simulink model "total_senario"  (R2019a)
settings: Solver=ode4  StartTime=0.0  StopTime=40  FixedStep=0.001  RelTol=1e-3
libraries: nesl_utility x16, sm_lib x13, simulink x1
(part 2 of 3)

== matlab function total_senario/SMC/MATLAB Function ==
  data: q input; u output; qd input; Dqd input; D2qd input
function u = fcn(q, qd, Dqd, D2qd)

c = 10;
k = 100;

L1 = 0.3; L2 = 0.4; L3 = 0.08;
c1 =  c; c2 = c; c3 = c; c4 = c;
k1 = k; k2 = k; k3 = k; k4 = k;
m1 = 4; m2 = 3; m3 = 1;

% s1 = 0;
% s2 = 0;
% s3 = 0;
% s4 = 0;

% SMC
e1 = qd(1) - q(1);
e2 = Dqd(1) - q(2);

e3 = qd(2) - q(3);
e4 = Dqd(2) - q(4);

e5 = qd(3) - q(5);
e6 = Dqd(3) - q(6);

e7 = qd(4) - q(7);
e8 = Dqd(4) - q(8);



s1 = c1*e1 + e2 ;
s2 = c2*e3 + e4 ;
s3 = c3*e5 + e6 ;
s4 = c4*e7 + e8 ;

%sgn
% if s1 > 0
%     sgn1 = 1;
% elseif s1 == 0
%     sgn1 = 0;
% elseif s1 < 0  
%     sgn1 = -1;
% end

% if s2 > 0
%     sgn2 = 1;
% elseif s2 == 0
%     sgn2 = 0;
% elseif s2 < 0  
%     sgn2 = -1;
% end

% if s3 > 0
%     sgn3 = 1;
% elseif s3 == 0
%     sgn3 = 0;
% elseif s3 < 0  
%     sgn3 = -1;
% end

% if s4 > 0
%     sgn4 = 1;
% elseif s4 == 0
%     sgn4 = 0;
% elseif s4 < 0  
%     sgn4 = -1;
% end

%sat
if abs(s1) <= 1
    sgn1 = s1;
elseif s1 > 1
    sgn1 = 1;
else
    sgn1 = -1;
end

if abs(s2) <= 1
    sgn2 = s2;
elseif s2 > 1
    sgn2 = 1;
else
    sgn2 = -1;
end

if abs(s3) <= 1
    sgn3 = s3;
elseif s3 > 1
    sgn3 = 1;
else
    sgn3 = -1;
end

if abs(s4) <= 1
    sgn4 = s4;
elseif s4 > 1
    sgn4 = 1;
else
    sgn4 = -1;
end

npsii = q(1);
ndpsii = q(2);
nth1 = q(3);
ndth1 = q(4);
nth2 = q(5);
ndth2 = q(6);
nth3 = q(7);
ndth3 = q(8);

%dynamcis
V = [- L3^2*m3*ndpsii*ndth1*sin(2*nth1 + 2*nth2 + 2*nth3) - L3^2*m3*ndpsii*ndth2*sin(2*nth1 + 2*nth2 + 2*nth3) - L3^2*m3*ndpsii*ndth3*sin(2*nth1 + 2*nth2 + 2*nth3) - L1^2*m1*ndpsii*ndth1*sin(2*nth1) - L1^2*m2*ndpsii*ndth1*sin(2*nth1) - L1^2*m3*ndpsii*ndth1*sin(2*nth1) - L2^2*m2*ndpsii*ndth1*sin(2*nth1 + 2*nth2) - L2^2*m2*ndpsii*ndth2*sin(2*nth1 + 2*nth2) - L2^2*m3*ndpsii*ndth1*sin(2*nth1 + 2*nth2) - L2^2*m3*ndpsii*ndth2*sin(2*nth1 + 2*nth2) - 2*L2*L3*m3*ndpsii*ndth1*sin(2*nth1 + 2*nth2 + nth3) - 2*L2*L3*m3*ndpsii*ndth2*sin(2*nth1 + 2*nth2 + nth3) - L2*L3*m3*ndpsii*ndth3*sin(2*nth1 + 2*nth2 + nth3) - L1*L2*m2*ndpsii*ndth2*sin(nth2) - L1*L2*m3*ndpsii*ndth2*sin(nth2) - L2*L3*m3*ndpsii*ndth3*sin(nth3) - 2*L1*L2*m2*ndpsii*ndth1*sin(2*nth1 + nth2) - L1*L2*m2*ndpsii*ndth2*sin(2*nth1 + nth2) - 2*L1*L2*m3*ndpsii*ndth1*sin(2*nth1 + nth2) - L1*L2*m3*ndpsii*ndth2*sin(2*nth1 + nth2) - 2*L1*L3*m3*ndpsii*ndth1*sin(2*nth1 + nth2 + nth3) - L1*L3*m3*ndpsii*ndth2*sin(2*nth1 + nth2 + nth3) - L1*L3*m3*ndpsii*ndth3*sin(2*nth1 + nth2 + nth3) - L1*L3*m3*ndpsii*ndth2*sin(nth2 + nth3) - L1*L3*m3*ndpsii*ndth3*sin(nth2 + nth3);
                                                                                                                                                                                                                                                                               (L3^2*m3*ndpsii^2*sin(2*nth1 + 2*nth2 + 2*nth3))/2 + (L1^2*m1*ndpsii^2*sin(2*nth1))/2 + (L1^2*m2*ndpsii^2*sin(2*nth1))/2 + (L1^2*m3*ndpsii^2*sin(2*nth1))/2 + (L2^2*m2*ndpsii^2*sin(2*nth1 + 2*nth2))/2 + (L2^2*m3*ndpsii^2*sin(2*nth1 + 2*nth2))/2 + L2*L3*m3*ndpsii^2*sin(2*nth1 + 2*nth2 + nth3) - L1*L2*m2*ndth2^2*sin(nth2) - L1*L2*m3*ndth2^2*sin(nth2) - L2*L3*m3*ndth3^2*sin(nth3) + L1*L2*m2*ndpsii^2*sin(2*nth1 + nth2) + L1*L2*m3*ndpsii^2*sin(2*nth1 + nth2) + L1*L3*m3*ndpsii^2*sin(2*nth1 + nth2 + nth3) - L1*L3*m3*ndth2^2*sin(nth2 + nth3) - L1*L3*m3*ndth3^2*sin(nth2 + nth3) - 2*L1*L2*m2*ndth1*ndth2*sin(nth2) - 2*L1*L2*m3*ndth1*ndth2*sin(nth2) - 2*L2*L3*m3*ndth1*ndth3*sin(nth3) - 2*L2*L3*m3*ndth2*ndth3*sin(nth3) - 2*L1*L3*m3*ndth1*ndth2*sin(nth2 + nth3) - 2*L1*L3*m3*ndth1*ndth3*sin(nth2 + nth3) - 2*L1*L3*m3*ndth2*ndth3*sin(nth2 + nth3);
                                                                                                                                                                                                                                                                                                                                                                                                                                                                                                       (L3^2*m3*ndpsii^2*sin(2*nth1 + 2*nth2 + 2*nth3))/2 + (L2^2*m2*ndpsii^2*sin(2*nth1 + 2*nth2))/2 + (L2^2*m3*ndpsii^2*sin(2*nth1 + 2*nth2))/2 + L2*L3*m3*ndpsii^2*sin(2*nth1 + 2*nth2 + nth3) + (L1*L2*m2*ndpsii^2*sin(nth2))/2 + (L1*L2*m3*ndpsii^2*sin(nth2))/2 + L1*L2*m2*ndth1^2*sin(nth2) + L1*L2*m3*ndth1^2*sin(nth2) - L2*L3*m3*ndth3^2*sin(nth3) + (L1*L2*m2*ndpsii^2*sin(2*nth1 + nth2))/2 + (L1*L2*m3*ndpsii^2*sin(2*nth1 + nth2))/2 + (L1*L3*m3*ndpsii^2*sin(2*nth1 + nth2 + nth3))/2 + (L1*L3*m3*ndpsii^2*sin(nth2 + nth3))/2 + L1*L3*m3*ndth1^2*sin(nth2 + nth3) - 2*L2*L3*m3*ndth1*ndth3*sin(nth3) - 2*L2*L3*m3*ndth2*ndth3*sin(nth3);
                                                                                                                                                                                                                                                                                                                                                                                                                                                                                                                                                                      (L3*m3*(L1*ndpsii^2*sin(nth2 + nth3) + 2*L1*ndth1^2*sin(nth2 + nth3) + L2*ndpsii^2*sin(2*nth1 + 2*nth2 + nth3) + L2*ndpsii^2*sin(nth3) + 2*L2*ndth1^2*sin(nth3) + 2*L2*ndth2^2*sin(nth3) + L3*ndpsii^2*sin(2*nth1 + 2*nth2 + 2*nth3) + L1*ndpsii^2*sin(2*nth1 + nth2 + nth3) + 2*L1*ndth1*ndth2*sin(nth2 + nth3) + 2*L1*ndth1*ndth3*sin(nth2 + nth3) + 4*L2*ndth1*ndth2*sin(nth3) + 2*L2*ndth1*ndth3*sin(nth3) + 2*L2*ndth2*ndth3*sin(nth3)))/2 - L3*m3*(L1*ndth1*ndth2*sin(nth2 + nth3) + L1*ndth1*ndth3*sin(nth2 + nth3) + L2*ndth1*ndth3*sin(nth3) + L2*ndth2*ndth3*sin(nth3))];
%
G = 9.81*[                                                                                                                                    0;
L3*m3*cos(nth1 + nth2 + nth3) + L2*m2*cos(nth1 + nth2) + L2*m3*cos(nth1 + nth2) + L1*m1*cos(nth1) + L1*m2*cos(nth1) + L1*m3*cos(nth1);
                                                      L3*m3*cos(nth1 + nth2 + nth3) + L2*m2*cos(nth1 + nth2) + L2*m3*cos(nth1 + nth2);
                                                                                                        L3*m3*cos(nth1 + nth2 + nth3)];
%
M = [[(L1^2*m1)/2 + (L1^2*m2)/2 + (L1^2*m3)/2 + (L2^2*m2)/2 + (L2^2*m3)/2 + (L3^2*m3)/2 + (L3^2*m3*cos(2*nth1 + 2*nth2 + 2*nth3))/2 + (L1^2*m1*cos(2*nth1))/2 + (L1^2*m2*cos(2*nth1))/2 + (L1^2*m3*cos(2*nth1))/2 + (L2^2*m2*cos(2*nth1 + 2*nth2))/2 + (L2^2*m3*cos(2*nth1 + 2*nth2))/2 + L1*L3*m3*cos(nth2 + nth3) + L2*L3*m3*cos(2*nth1 + 2*nth2 + nth3) + L1*L2*m2*cos(nth2) + L1*L2*m3*cos(nth2) + L2*L3*m3*cos(nth3) + L1*L2*m2*cos(2*nth1 + nth2) + L1*L2*m3*cos(2*nth1 + nth2) + L1*L3*m3*cos(2*nth1 + nth2 + nth3),                                                                                                                                                            0,                                                                                                                        0,                                                        0];
[                                                                                                                                                                                                                                                                                                                                                                                                                                                                                                                   0, L1^2*m1 + L1^2*m2 + L1^2*m3 + L2^2*m2 + L2^2*m3 + L3^2*m3 + 2*L1*L3*m3*cos(nth2 + nth3) + 2*L1*L2*m2*cos(nth2) + 2*L1*L2*m3*cos(nth2) + 2*L2*L3*m3*cos(nth3), L2^2*m2 + L2^2*m3 + L3^2*m3 + L1*L3*m3*cos(nth2 + nth3) + L1*L2*m2*cos(nth2) + L1*L2*m3*cos(nth2) + 2*L2*L3*m3*cos(nth3), L3^2*m3 + L1*L3*m3*cos(nth2 + nth3) + L2*L3*m3*cos(nth3)];
[                                                                                                                                                                                                                                                                                                                                                                                                                                                                                                                   0,                                     L2^2*m2 + L2^2*m3 + L3^2*m3 + L1*L3*m3*cos(nth2 + nth3) + L1*L2*m2*cos(nth2) + L1*L2*m3*cos(nth2) + 2*L2*L3*m3*cos(nth3),                                                                       L2^2*m2 + L2^2*m3 + L3^2*m3 + 2*L2*L3*m3*cos(nth3),                             m3*L3^2 + L2*m3*cos(nth3)*L3];
[                                                                                                                                                                                                                                                                                                                                                                                                                                                                                                                   0,                                                                                                              L3*m3*(L3 + L1*cos(nth2 + nth3) + L2*cos(nth3)),                                                                                                L3*m3*(L3 + L2*cos(nth3)),                                                  L3^2*m3]];
%

N = V + G;

F = -pinv(M)*N ;

% X(1) = psi, X(3) = th1, X(5) = th2, X(7) = th3
tau1_hat = c1*e2 + D2qd(1) - F(1) + k1*sgn1 ;
tau2_hat = c2*e4 + D2qd(2) - F(2) + k2*sgn2 ;
tau3_hat = c3*e6 + D2qd(3) - F(3) + k3*sgn3 ;
tau4_hat = c4*e8 + D2qd(4) - F(4) + k4*sgn4 ;

Tau_hat = [tau1_hat;tau2_hat;tau3_hat;tau4_hat];

u = M*[tau1_hat;tau2_hat;tau3_hat;tau4_hat] ;
% tau1 = u(1) ;
% tau2 = u(2) ;
% tau3 = u(3) ;
% tau4 = u(4) ;

% x_ddt = pinv(M)*(Tau_hat - N) ;
% x_ddt = pinv(M)*(Tau - N) ;


% if abs(e1*e2) < 0.05
%     t_reg1 = t;
% else
%     t_reg1 = 0;
% end
% 
% if abs(e3*e4) < 0.05
%     t_reg2 = t;
% else
%     t_reg2 = 0;
% end
% 
% if abs(e5*e6) < 0.05
%     t_reg3 = t;
% else
%     t_reg3 = 0;
% end
% 
% if abs(e7*e8) < 0.05
%     t_reg4 = t;
% else
%     t_reg4 = 0;
% end

% dXdt = [X(2); x_ddt(1) ; X(4); x_ddt(2); X(6); x_ddt(3); X(8); x_ddt(4) ] ;
end


%%%%%%%%%%%%%%%%%%%%%%%%%%%%%%%%%%%%%%%%%%%%%%%%%%%%%%%%%%%%%%%%%%%%%%%%%%%%%%%%%%%%%%%%%%%%%%%%
% function u = fcn(q, qd, Dqd, D2qd)
% u = zeros(4, 1);
% 
% % parameter
% g = 9.81;
% m1 = 4;
% m2 = 3;
% m3 = 1;
% L1 = 0.4;
% L2 = 0.3;
% L3 = 0.08;
% 
% npsii = q(1);
% nth1 = q(2);
% nth2 = q(3);
% nth3 = q(4);
% ndpsii = q(5);
% ndth1 = q(6);
% ndth2 = q(7);
% ndth3 = q(8);
% 
% 
% M11 = (L1^2*m1)/2 + (L1^2*m2)/2 + (L1^2*m3)/2 + (L2^2*m2)/2 + (L2^2*m3)/2 + (L3^2*m3)/2 + (L3^2*m3*cos(2*nth1 + 2*nth2 + 2*nth3))/2 + (L1^2*m1*cos(2*nth1))/2 + (L1^2*m2*cos(2*nth1))/2 + (L1^2*m3*cos(2*nth1))/2 + (L2^2*m2*cos(2*nth1 + 2*nth2))/2 + (L2^2*m3*cos(2*nth1 + 2*nth2))/2 + L1*L3*m3*cos(nth2 + nth3) + L2*L3*m3*cos(2*nth1 + 2*nth2 + nth3) + L1*L2*m2*cos(nth2) + L1*L2*m3*cos(nth2) + L2*L3*m3*cos(nth3) + L1*L2*m2*cos(2*nth1 + nth2) + L1*L2*m3*cos(2*nth1 + nth2) + L1*L3*m3*cos(2*nth1 + nth2 + nth3);
% M12 = 0;
% M13 = 0;
% M14 = 0;
% 
% M21 = 0;
% M22 = L1^2*m1 + L1^2*m2 + L1^2*m3 + L2^2*m2 + L2^2*m3 + L3^2*m3 + 2*L1*L3*m3*cos(nth2 + nth3) + 2*L1*L2*m2*cos(nth2) + 2*L1*L2*m3*cos(nth2) + 2*L2*L3*m3*cos(nth3);
% M23 = L2^2*m2 + L2^2*m3 + L3^2*m3 + L1*L3*m3*cos(nth2 + nth3) + L1*L2*m2*cos(nth2) + L1*L2*m3*cos(nth2) + 2*L2*L3*m3*cos(nth3);
% M24 = L3^2*m3 + L1*L3*m3*cos(nth2 + nth3) + L2*L3*m3*cos(nth3);
% 
% M31 = 0;
% M32 = L2^2*m2 + L2^2*m3 + L3^2*m3 + L1*L3*m3*cos(nth2 + nth3) + L1*L2*m2*cos(nth2) + L1*L2*m3*cos(nth2) + 2*L2*L3*m3*cos(nth3);
% M33 = L2^2*m2 + L2^2*m3 + L3^2*m3 + 2*L2*L3*m3*cos(nth3);
% M34 = m3*L3^2 + L2*m3*cos(nth3)*L3;
% 
% M41 = 0;
% M42 = L3*m3*(L3 + L1*cos(nth2 + nth3) + L2*cos(nth3));
% M43 = L3*m3*(L3 + L2*cos(nth3));
% M44 = L3^2*m3;
% 
% M = [M11 M12 M13 M14; M21 M22 M23 M24 ;M31 M32 M33 M34 ;M41 M42 M43 M44];
% 
% % coriolis vector, [V]
% V1 = -L3^2*m3*ndpsii*ndth1*sin(2*nth1 + 2*nth2 + 2*nth3) - L3^2*m3*ndpsii*ndth2*sin(2*nth1 + 2*nth2 + 2*nth3) - L3^2*m3*ndpsii*ndth3*sin(2*nth1 + 2*nth2 + 2*nth3) - L1^2*m1*ndpsii*ndth1*sin(2*nth1) - L1^2*m2*ndpsii*ndth1*sin(2*nth1) - L1^2*m3*ndpsii*ndth1*sin(2*nth1) - L2^2*m2*ndpsii*ndth1*sin(2*nth1 + 2*nth2) - L2^2*m2*ndpsii*ndth2*sin(2*nth1 + 2*nth2) - L2^2*m3*ndpsii*ndth1*sin(2*nth1 + 2*nth2) - L2^2*m3*ndpsii*ndth2*sin(2*nth1 + 2*nth2) - 2*L2*L3*m3*ndpsii*ndth1*sin(2*nth1 + 2*nth2 + nth3) - 2*L2*L3*m3*ndpsii*ndth2*sin(2*nth1 + 2*nth2 + nth3) - L2*L3*m3*ndpsii*ndth3*sin(2*nth1 + 2*nth2 + nth3) - L1*L2*m2*ndpsii*ndth2*sin(nth2) - L1*L2*m3*ndpsii*ndth2*sin(nth2) - L2*L3*m3*ndpsii*ndth3*sin(nth3) - 2*L1*L2*m2*ndpsii*ndth1*sin(2*nth1 + nth2) - L1*L2*m2*ndpsii*ndth2*sin(2*nth1 + nth2) - 2*L1*L2*m3*ndpsii*ndth1*sin(2*nth1 + nth2) - L1*L2*m3*ndpsii*ndth2*sin(2*nth1 + nth2) - 2*L1*L3*m3*ndpsii*ndth1*sin(2*nth1 + nth2 + nth3) - L1*L3*m3*ndpsii*ndth2*sin(2*nth1 + nth2 + nth3) - L1*L3*m3*ndpsii*ndth3*sin(2*nth1 + nth2 + nth3) - L1*L3*m3*ndpsii*ndth2*sin(nth2 + nth3) - L1*L3*m3*ndpsii*ndth3*sin(nth2 + nth3);
% V2 = (L3^2*m3*ndpsii^2*sin(2*nth1 + 2*nth2 + 2*nth3))/2 + (L1^2*m1*ndpsii^2*sin(2*nth1))/2 + (L1^2*m2*ndpsii^2*sin(2*nth1))/2 + (L1^2*m3*ndpsii^2*sin(2*nth1))/2 + (L2^2*m2*ndpsii^2*sin(2*nth1 + 2*nth2))/2 + (L2^2*m3*ndpsii^2*sin(2*nth1 + 2*nth2))/2 + L2*L3*m3*ndpsii^2*sin(2*nth1 + 2*nth2 + nth3) - L1*L2*m2*ndth2^2*sin(nth2) - L1*L2*m3*ndth2^2*sin(nth2) - L2*L3*m3*ndth3^2*sin(nth3) + L1*L2*m2*ndpsii^2*sin(2*nth1 + nth2) + L1*L2*m3*ndpsii^2*sin(2*nth1 + nth2) + L1*L3*m3*ndpsii^2*sin(2*nth1 + nth2 + nth3) - L1*L3*m3*ndth2^2*sin(nth2 + nth3) - L1*L3*m3*ndth3^2*sin(nth2 + nth3) - 2*L1*L2*m2*ndth1*ndth2*sin(nth2) - 2*L1*L2*m3*ndth1*ndth2*sin(nth2) - 2*L2*L3*m3*ndth1*ndth3*sin(nth3) - 2*L2*L3*m3*ndth2*ndth3*sin(nth3) - 2*L1*L3*m3*ndth1*ndth2*sin(nth2 + nth3) - 2*L1*L3*m3*ndth1*ndth3*sin(nth2 + nth3) - 2*L1*L3*m3*ndth2*ndth3*sin(nth2 + nth3);
% V3 = (L3^2*m3*ndpsii^2*sin(2*nth1 + 2*nth2 + 2*nth3))/2 + (L2^2*m2*ndpsii^2*sin(2*nth1 + 2*nth2))/2 + (L2^2*m3*ndpsii^2*sin(2*nth1 + 2*nth2))/2 + L2*L3*m3*ndpsii^2*sin(2*nth1 + 2*nth2 + nth3) + (L1*L2*m2*ndpsii^2*sin(nth2))/2 + (L1*L2*m3*ndpsii^2*sin(nth2))/2 + L1*L2*m2*ndth1^2*sin(nth2) + L1*L2*m3*ndth1^2*sin(nth2) - L2*L3*m3*ndth3^2*sin(nth3) + (L1*L2*m2*ndpsii^2*sin(2*nth1 + nth2))/2 + (L1*L2*m3*ndpsii^2*sin(2*nth1 + nth2))/2 + (L1*L3*m3*ndpsii^2*sin(2*nth1 + nth2 + nth3))/2 + (L1*L3*m3*ndpsii^2*sin(nth2 + nth3))/2 + L1*L3*m3*ndth1^2*sin(nth2 + nth3) - 2*L2*L3*m3*ndth1*ndth3*sin(nth3) - 2*L2*L3*m3*ndth2*ndth3*sin(nth3);
% V4 = (L3*m3*(L1*ndpsii^2*sin(nth2 + nth3) + 2*L1*ndth1^2*sin(nth2 + nth3) + L2*ndpsii^2*sin(2*nth1 + 2*nth2 + nth3) + L2*ndpsii^2*sin(nth3) + 2*L2*ndth1^2*sin(nth3) + 2*L2*ndth2^2*sin(nth3) + L3*ndpsii^2*sin(2*nth1 + 2*nth2 + 2*nth3) + L1*ndpsii^2*sin(2*nth1 + nth2 + nth3) + 2*L1*ndth1*ndth2*sin(nth2 + nth3) + 2*L1*ndth1*ndth3*sin(nth2 + nth3) + 4*L2*ndth1*ndth2*sin(nth3) + 2*L2*ndth1*ndth3*sin(nth3) + 2*L2*ndth2*ndth3*sin(nth3)))/2 - L3*m3*(L1*ndth1*ndth2*sin(nth2 + nth3) + L1*ndth1*ndth3*sin(nth2 + nth3) + L2*ndth1*ndth3*sin(nth3) + L2*ndth2*ndth3*sin(nth3));
% 
% V = [V1; V2; V3; V4];
% 
% % gravity vector, [G]
% G1 = 0;
% G2 = g*(L3*m3*cos(nth1 + nth2 + nth3) + L2*m2*cos(nth1 + nth2) + L2*m3*cos(nth1 + nth2) + L1*m1*cos(nth1) + L1*m2*cos(nth1) + L1*m3*cos(nth1));
% G3 = g*(L3*m3*cos(nth1 + nth2 + nth3) + L2*m2*cos(nth1 + nth2) + L2*m3*cos(nth1 + nth2));
% G4 = L3*g*m3*cos(nth1 + nth2 + nth3);
% 
% G = [G1; G2; G3; G4];
% 
% % SMC
% e1 = qd(1) - q(1);
% e2 = qd(2) - q(2);
% e3 = qd(3) - q(3);
% e4 = qd(4) - q(4);
% 
% e5 = Dqd(1) - q(5);
% e6 = Dqd(2) - q(6);
% e7 = Dqd(3) - q(7);
% e8 = Dqd(4) - q(8);
% 
% % [C] matrix
% c1 = 5;
% c2 = 5;
% c3 = 5;
% c4 = 5;
% C = diag([c1, c2, c3, c4]);
% 
% % sliding line
% s = [e5; e6; e7; e8] + C*[e1; e2; e3; e4];
% 
% % design [Q], [K]
% del1 = 0.005*10^4;
% del2 = 0.005*10^4;
% del3 = 0.005*10^4;
% del4 = 0.005*10^4;
% 
% A = M\eye(size(M));
% w1max = abs(A(1, 1))*del1 + abs(A(1, 2))*del2 + abs(A(1, 3))*del3 + abs(A(1,4))*del4;
% w2max = abs(A(2, 1))*del1 + abs(A(2, 2))*del2 + abs(A(2, 3))*del3 + abs(A(2,4))*del4;
% w3max = abs(A(3, 1))*del1 + abs(A(3, 2))*del2 + abs(A(3, 3))*del3 + abs(A(3,4))*del4;
% w4max = abs(A(4, 1))*del1 + abs(A(4, 2))*del2 + abs(A(4, 3))*del3 + abs(A(4,4))*del4;
% 
% k1 = 5;
% k2 = 5;
% k3 = 5;
% k4 = 5;
% 
% Q1 = -k1 - w1max;
% Q2 = -k2 - w2max;
% Q3 = -k3 - w3max;
% Q4 = -k4 - w4max;
% 
% Q = diag([Q1, Q2, Q3, Q4]);
% K = M*Q;
% u_eq = M*[D2qd(1); D2qd(2); D2qd(3); D2qd(4)] + M*C*[e5; e6; e7; e8] + V + G;
% 
% eps = 1;
% if (abs(s(1)) < eps)
%     sat_s1 = s(1)/eps;
% else
%     sat_s1 = sign(s(1));
% end
%     
% if (abs(s(2)) < eps)
%     sat_s2 = s(2)/eps;
% else
%     sat_s2 = sign(s(2));
% end
%     
% if (abs(s(3)) < eps)
%     sat_s3 = s(3)/eps;
% else
%     sat_s3 = sign(s(3));
% end
%     
% if (abs(s(4)) < eps)
%     sat_s4 = s(4)/eps;
% else
%     sat_s4 = sign(s(4));
% end
% u = u_eq - K*[sat_s1; sat_s2; sat_s3; sat_s4];

== matlab function total_senario/Desired Joint Trajectory/MATLAB Function ==
  data: u input; qd output

function qd = fcn(u)
t = u(1);
% time = 0:0.01:10

% (1) r_t,theta_t _ // for Tornado
% cycle=5; % 해당 시간동안 몇바퀴 돌지_진동수
% r_t = 0.1 - (0.1/tf)*t; 
% w_t = cycle*2*pi/tf; 
% theta_t = w_t*t;
% 
% % (2) waffle 중심 cartesian coordinate
% x_wa = r_t.*cos(theta_t); % waffle 중심  
% y_wa = r_t.*sin(theta_t) + 0.4;
% z_wa = - 0.2 - (0.3/tf)*t + 0.6; 
% r_wa = sqrt(x_wa.^2+y_wa.^2);

% psii= atan2(y_wa,x_wa);
% th2 = acos((r_wa.^2+z_wa.^2-L1^2-L2^2)./(2*L1*L2)); % r,z 좌표계로 사이드뷰
% th1 = atan2(z_wa-L3,r_wa) - atan2(L2*sin(th2),L1+L2*cos(th2));
% th3 = pi/2-th1-th2;

x = 0;
y = 0.4;

scale_factor = 1/80;
cycle = 1;
time = 1; %% 20
t=t/time;
w = 2*pi*cycle;
theta = w*t;


psii= psid(t);
th2 = th2d(t); % r,z 좌표계로 사이드뷰
th1 = th1d(t);
th3 = th3d(t);


qd = [psii; th1; th2; th3];

end

function y = s(t)
% if (-1<=t && t<3)
%     y = 2/3*t^3 - 8/27*t^4 +1/27*t^5;
% %     y = 3/2*t^3 - 1*t^4 +3/16*t^5; % 5 / 2
% %     y = 6*t^3 -8*t^4 + 3*t^5; % 5차 1초
% %     y = 2/3*t^2-1/9*t^3; % 3초
% %     y = t^2 - 0.25*t^3; % 2초
% %     y = 2*t^2 - t^3; % 1초
% %     y = t^2;
% elseif (3<=t && t<7)
%     y = t;
% elseif (7<=t &&  t<=10.01)
%     y = -37730/27 + 2600/3*t -5740/27*t^2 + 698/27*t^3 -14/9*t^4 + 1/27*t^5;
% %     y = -10240 + 5825*t -1320*t^2 + 149*t^3 -67/8*t^4 + 3/16*t^5; % 5 / 2
% %     y = -225990 + 119800*t -25380*t^2 + 2686*t^3 -142*t^4 + 3*t^5; % 5차1s
% %     y = 490/9 - 20*t + 8/3*t^2 - 1/9*t^3; % 3초
% %     y = 160 - 55*t +6.5 * t^2 - 0.25*t^3; % 2초
% %     y = 810 - 260*t + 28*t^2 - t^3; % 1초
% %     y = 10 - (t-10)^2;
% else
%     y=t;
% end
y = t;
end


function q = psid(t)

% global L1 L2 L3;
% q = 1.32;
q = atan2(yd(t),xd(t));
% q = 1.32;
end

function q = th1d(t)
L0=1.5;L1=0.3;L2=0.3;L3=0.08; % L3 항상 지면에 수직. 
tf=10; w = 10*pi/tf;
% global L1 L2 L3;
% q = -pi/6;
q = atan2(zd(t)-L3-1.5,sqrt(xd(t)^2+yd(t)^2)) - atan2(L2*sin(th2d(t)),L1+L2*cos(th2d(t)));
% q = -1.52;
end

function q = th2d(t)
L0=1.5;L1=0.3;L2=0.3;L3=0.08; % L3 항상 지면에 수직. 
tf=10; w = 10*pi/tf;
% global L1 L2 L3;
% q = pi/3;
q = acos((xd(t)^2 + yd(t)^2 +(zd(t)-L3-1.5)^2-L1^2-L2^2)/(2*L1*L2));
% q = 1.57;
end

function y = th3d(t)
L0=1.5;L1=0.3;L2=0.3;L3=0.08; % L3 항상 지면에 수직. 
tf=10; w = 10*pi/tf;
% global L1 L2 L3;
y = pi/2 - th1d(t) - th2d(t);
% y = 1.52;
end

function y = xd(t)
L0=1.5;L1=0.3;L2=0.3;L3=0.08; % L3 항상 지면에 수직.
scale_factor = 1/80; cycle = 1;
tf=10; w = 2*pi*cycle;
y = scale_factor*8*cos(w*s(t))- 1.469294361278199e-06;
% global L1 L2 L3 w tf;
% y = ((10 - (10/tf)*(t))*cos(w*(t)))/100;
% y = ((10 - (10/tf)*s(t))*cos(w*s(t)))/100;
% y = (50*cos(pi/4)+(-2*50*cos(pi/4))*s(t)/tf)/100; % 서빙 to 어피치 
end

function y = yd(t)
L0=1.5;L1=0.3;L2=0.3;L3=0.08; % L3 항상 지면에 수직. 
scale_factor = 1/80; cycle = 1;
tf=10; w = 2*pi*cycle;
y = scale_factor*8*sin(w*s(t)) + 0.4+ 0.00000326818465700;
% global L1 L2 L3 w tf;
% y = ((10 - (10/tf)*(t))*sin(w*(t)) + 40)/100;  % (0,40) 에서 sprial sink./*
% y = ((10 - (10/tf)*s(t))*sin(w*s(t)) + 40)/100;  % (0,40) 에서 sprial sink.
% y = (0.7 .* s(t).*(s(t)-10) + 50*sin(pi/4))/100; % 두배가량 내려감
end

function y = zd(t)
L0=1.5;L1=0.3;L2=0.3;L3=0.08; % L3 항상 지면에 수직. 
scale_factor = 1/80; cycle = 1;
tf=10; w = 2*pi*cycle;
y = 1.3+ 0.000013186867988;
end

== matlab function total_senario/Desired Joint Trajectory/MATLAB Function2 ==
  data: u input; qd output

function qd = fcn(u)
t = u(1);
% time = 0:0.01:10

% (1) r_t,theta_t _ // for Tornado
% cycle=5; % 해당 시간동안 몇바퀴 돌지_진동수
% r_t = 0.1 - (0.1/tf)*t; 
% w_t = cycle*2*pi/tf; 
% theta_t = w_t*t;
% 
% % (2) waffle 중심 cartesian coordinate
% x_wa = r_t.*cos(theta_t); % waffle 중심  
% y_wa = r_t.*sin(theta_t) + 0.4;
% z_wa = - 0.2 - (0.3/tf)*t + 0.6; 
% r_wa = sqrt(x_wa.^2+y_wa.^2);

% psii= atan2(y_wa,x_wa);
% th2 = acos((r_wa.^2+z_wa.^2-L1^2-L2^2)./(2*L1*L2)); % r,z 좌표계로 사이드뷰
% th1 = atan2(z_wa-L3,r_wa) - atan2(L2*sin(th2),L1+L2*cos(th2));
% th3 = pi/2-th1-th2;

x = 0;
y = 0.4;

scale_factor = 1/80;
cycle = 1;
time = 1; %% 20
t=t/time;
w = 2*pi*cycle;
theta = w*t;


psii= psid(t);
th2 = th2d(t); % r,z 좌표계로 사이드뷰
th1 = th1d(t);
th3 = th3d(t);


qd = [psii; th1; th2; th3];

end

function y = s(t)
% if (-1<=t && t<3)
%     y = 2/3*t^3 - 8/27*t^4 +1/27*t^5;
% %     y = 3/2*t^3 - 1*t^4 +3/16*t^5; % 5 / 2
% %     y = 6*t^3 -8*t^4 + 3*t^5; % 5차 1초
% %     y = 2/3*t^2-1/9*t^3; % 3초
% %     y = t^2 - 0.25*t^3; % 2초
% %     y = 2*t^2 - t^3; % 1초
% %     y = t^2;
% elseif (3<=t && t<7)
%     y = t;
% elseif (7<=t &&  t<=10.01)
%     y = -37730/27 + 2600/3*t -5740/27*t^2 + 698/27*t^3 -14/9*t^4 + 1/27*t^5;
% %     y = -10240 + 5825*t -1320*t^2 + 149*t^3 -67/8*t^4 + 3/16*t^5; % 5 / 2
% %     y = -225990 + 119800*t -25380*t^2 + 2686*t^3 -142*t^4 + 3*t^5; % 5차1s
% %     y = 490/9 - 20*t + 8/3*t^2 - 1/9*t^3; % 3초
% %     y = 160 - 55*t +6.5 * t^2 - 0.25*t^3; % 2초
% %     y = 810 - 260*t + 28*t^2 - t^3; % 1초
% %     y = 10 - (t-10)^2;
% else
%     y=t;
% end
y = t;
end


function q = psid(t)

% global L1 L2 L3;
% q = 1.32;
q = atan2(yd(t),xd(t));
% q = 1.32;
end

function q = th1d(t)
L0=1.5;L1=0.3;L2=0.3;L3=0.08; % L3 항상 지면에 수직. 
tf=10; w = 10*pi/tf;
% global L1 L2 L3;
% q = -pi/6;
q = atan2(zd(t)-L3-1.5,sqrt(xd(t)^2+yd(t)^2)) - atan2(L2*sin(th2d(t)),L1+L2*cos(th2d(t)));
% q = -1.52;
end

function q = th2d(t)
L0=1.5;L1=0.3;L2=0.3;L3=0.08; % L3 항상 지면에 수직. 
tf=10; w = 10*pi/tf;
% global L1 L2 L3;
% q = pi/3;
q = acos((xd(t)^2 + yd(t)^2 +(zd(t)-L3-1.5)^2-L1^2-L2^2)/(2*L1*L2));
% q = 1.57;
end

function y = th3d(t)
L0=1.5;L1=0.3;L2=0.3;L3=0.08; % L3 항상 지면에 수직. 
tf=10; w = 10*pi/tf;
% global L1 L2 L3;
y = pi/2 - th1d(t) - th2d(t);
% y = 1.52;
end

function y = xd(t)
L0=1.5;L1=0.3;L2=0.3;L3=0.08; % L3 항상 지면에 수직.
scale_factor = 1/80; cycle = 1;
tf=10; w = 2*pi*cycle;
y = scale_factor*(-6 + cos(w*s(t)))-4.1750e-04- 1.469294361278199e-06;
% global L1 L2 L3 w tf;
% y = ((10 - (10/tf)*(t))*cos(w*(t)))/100;
% y = ((10 - (10/tf)*s(t))*cos(w*s(t)))/100;
% y = (50*cos(pi/4)+(-2*50*cos(pi/4))*s(t)/tf)/100; % 서빙 to 어피치 
end

function y = yd(t)
L0=1.5;L1=0.3;L2=0.3;L3=0.08; % L3 항상 지면에 수직. 
scale_factor = 1/80; cycle = 1;
tf=10; w = 2*pi*cycle;
y = scale_factor*(6 + sin(w*s(t))) + 0.4-1.0582e-04+ 0.00000326818465700;
% global L1 L2 L3 w tf;
% y = ((10 - (10/tf)*(t))*sin(w*(t)) + 40)/100;  % (0,40) 에서 sprial sink./*
% y = ((10 - (10/tf)*s(t))*sin(w*s(t)) + 40)/100;  % (0,40) 에서 sprial sink.
% y = (0.7 .* s(t).*(s(t)-10) + 50*sin(pi/4))/100; % 두배가량 내려감
end

function y = zd(t)
L0=1.5;L1=0.3;L2=0.3;L3=0.08; % L3 항상 지면에 수직. 
scale_factor = 1/80; cycle = 1;
tf=10; w = 2*pi*cycle;
y = 1.3+ 0.000013186867988;
end

== matlab function total_senario/Desired Joint Trajectory/MATLAB Function3 ==
  data: u input; qd output

function qd = fcn(u)
t = u(1);
% time = 0:0.01:10

% (1) r_t,theta_t _ // for Tornado
% cycle=5; % 해당 시간동안 몇바퀴 돌지_진동수
% r_t = 0.1 - (0.1/tf)*t; 
% w_t = cycle*2*pi/tf; 
% theta_t = w_t*t;
% 
% % (2) waffle 중심 cartesian coordinate
% x_wa = r_t.*cos(theta_t); % waffle 중심  
% y_wa = r_t.*sin(theta_t) + 0.4;
% z_wa = - 0.2 - (0.3/tf)*t + 0.6; 
% r_wa = sqrt(x_wa.^2+y_wa.^2);

% psii= atan2(y_wa,x_wa);
% th2 = acos((r_wa.^2+z_wa.^2-L1^2-L2^2)./(2*L1*L2)); % r,z 좌표계로 사이드뷰
% th1 = atan2(z_wa-L3,r_wa) - atan2(L2*sin(th2),L1+L2*cos(th2));
% th3 = pi/2-th1-th2;

x = 0;
y = 0.4;

scale_factor = 1/80;
cycle = 1;
time = 1; %% 20
t=t/time;
w = 2*pi*cycle;
theta = w*t;


psii= psid(t);
th2 = th2d(t); % r,z 좌표계로 사이드뷰
th1 = th1d(t);
th3 = th3d(t);


qd = [psii; th1; th2; th3];

end

function y = s(t)
% if (-1<=t && t<3)
%     y = 2/3*t^3 - 8/27*t^4 +1/27*t^5;
% %     y = 3/2*t^3 - 1*t^4 +3/16*t^5; % 5 / 2
% %     y = 6*t^3 -8*t^4 + 3*t^5; % 5차 1초
% %     y = 2/3*t^2-1/9*t^3; % 3초
% %     y = t^2 - 0.25*t^3; % 2초
% %     y = 2*t^2 - t^3; % 1초
% %     y = t^2;
% elseif (3<=t && t<7)
%     y = t;
% elseif (7<=t &&  t<=10.01)
%     y = -37730/27 + 2600/3*t -5740/27*t^2 + 698/27*t^3 -14/9*t^4 + 1/27*t^5;
% %     y = -10240 + 5825*t -1320*t^2 + 149*t^3 -67/8*t^4 + 3/16*t^5; % 5 / 2
% %     y = -225990 + 119800*t -25380*t^2 + 2686*t^3 -142*t^4 + 3*t^5; % 5차1s
% %     y = 490/9 - 20*t + 8/3*t^2 - 1/9*t^3; % 3초
% %     y = 160 - 55*t +6.5 * t^2 - 0.25*t^3; % 2초
% %     y = 810 - 260*t + 28*t^2 - t^3; % 1초
% %     y = 10 - (t-10)^2;
% else
%     y=t;
% end
y = t;
end


function q = psid(t)

% global L1 L2 L3;
% q = 1.32;
q = atan2(yd(t),xd(t));
% q = 1.32;
end

function q = th1d(t)
L0=1.5;L1=0.3;L2=0.3;L3=0.08; % L3 항상 지면에 수직. 
tf=10; w = 10*pi/tf;
% global L1 L2 L3;
% q = -pi/6;
q = atan2(zd(t)-L3-1.5,sqrt(xd(t)^2+yd(t)^2)) - atan2(L2*sin(th2d(t)),L1+L2*cos(th2d(t)));
% q = -1.52;
end

function q = th2d(t)
L0=1.5;L1=0.3;L2=0.3;L3=0.08; % L3 항상 지면에 수직. 
tf=10; w = 10*pi/tf;
% global L1 L2 L3;
% q = pi/3;
q = acos((xd(t)^2 + yd(t)^2 +(zd(t)-L3-1.5)^2-L1^2-L2^2)/(2*L1*L2));
% q = 1.57;
end

function y = th3d(t)
L0=1.5;L1=0.3;L2=0.3;L3=0.08; % L3 항상 지면에 수직. 
tf=10; w = 10*pi/tf;
% global L1 L2 L3;
y = pi/2 - th1d(t) - th2d(t);
% y = 1.52;
end

function y = xd(t)
L0=1.5;L1=0.3;L2=0.3;L3=0.08; % L3 항상 지면에 수직.
scale_factor = 1/80; cycle = 1;
tf=10; w = 2*pi*cycle;
y = scale_factor*(-1 + cos(w*s(t)))-4.1750e-04- 1.469294361278199e-06;
% global L1 L2 L3 w tf;
% y = ((10 - (10/tf)*(t))*cos(w*(t)))/100;
% y = ((10 - (10/tf)*s(t))*cos(w*s(t)))/100;
% y = (50*cos(pi/4)+(-2*50*cos(pi/4))*s(t)/tf)/100; % 서빙 to 어피치 
end

function y = yd(t)
L0=1.5;L1=0.3;L2=0.3;L3=0.08; % L3 항상 지면에 수직. 
scale_factor = 1/80; cycle = 1;
tf=10; w = 2*pi*cycle;
y = scale_factor*(-2 + sin(w*s(t))) + 0.4-1.0582e-04+ 0.00000326818465700;
% global L1 L2 L3 w tf;
% y = ((10 - (10/tf)*(t))*sin(w*(t)) + 40)/100;  % (0,40) 에서 sprial sink./*
% y = ((10 - (10/tf)*s(t))*sin(w*s(t)) + 40)/100;  % (0,40) 에서 sprial sink.
% y = (0.7 .* s(t).*(s(t)-10) + 50*sin(pi/4))/100; % 두배가량 내려감
end

function y = zd(t)
L0=1.5;L1=0.3;L2=0.3;L3=0.08; % L3 항상 지면에 수직. 
scale_factor = 1/80; cycle = 1;
tf=10; w = 2*pi*cycle;
y = 1.3+ 0.000013186867988;
end

== matlab function total_senario/Desired Joint Trajectory/MATLAB Function4 ==
  data: u input; qd output

function qd = fcn(u)
t = u(1);
% time = 0:0.01:10

% (1) r_t,theta_t _ // for Tornado
% cycle=5; % 해당 시간동안 몇바퀴 돌지_진동수
% r_t = 0.1 - (0.1/tf)*t; 
% w_t = cycle*2*pi/tf; 
% theta_t = w_t*t;
% 
% % (2) waffle 중심 cartesian coordinate
% x_wa = r_t.*cos(theta_t); % waffle 중심  
% y_wa = r_t.*sin(theta_t) + 0.4;
% z_wa = - 0.2 - (0.3/tf)*t + 0.6; 
% r_wa = sqrt(x_wa.^2+y_wa.^2);

% psii= atan2(y_wa,x_wa);
% th2 = acos((r_wa.^2+z_wa.^2-L1^2-L2^2)./(2*L1*L2)); % r,z 좌표계로 사이드뷰
% th1 = atan2(z_wa-L3,r_wa) - atan2(L2*sin(th2),L1+L2*cos(th2));
% th3 = pi/2-th1-th2;

x = 0;
y = 0.4;

scale_factor = 1/80;
cycle = 1;
time = 1; %% 20
t=t/time;
w = 2*pi*cycle;
theta = w*t;


psii= psid(t);
th2 = th2d(t); % r,z 좌표계로 사이드뷰
th1 = th1d(t);
th3 = th3d(t);


qd = [psii; th1; th2; th3];

end

function y = s(t)
% if (-1<=t && t<3)
%     y = 2/3*t^3 - 8/27*t^4 +1/27*t^5;
% %     y = 3/2*t^3 - 1*t^4 +3/16*t^5; % 5 / 2
% %     y = 6*t^3 -8*t^4 + 3*t^5; % 5차 1초
% %     y = 2/3*t^2-1/9*t^3; % 3초
% %     y = t^2 - 0.25*t^3; % 2초
% %     y = 2*t^2 - t^3; % 1초
% %     y = t^2;
% elseif (3<=t && t<7)
%     y = t;
% elseif (7<=t &&  t<=10.01)
%     y = -37730/27 + 2600/3*t -5740/27*t^2 + 698/27*t^3 -14/9*t^4 + 1/27*t^5;
% %     y = -10240 + 5825*t -1320*t^2 + 149*t^3 -67/8*t^4 + 3/16*t^5; % 5 / 2
% %     y = -225990 + 119800*t -25380*t^2 + 2686*t^3 -142*t^4 + 3*t^5; % 5차1s
% %     y = 490/9 - 20*t + 8/3*t^2 - 1/9*t^3; % 3초
% %     y = 160 - 55*t +6.5 * t^2 - 0.25*t^3; % 2초
% %     y = 810 - 260*t + 28*t^2 - t^3; % 1초
% %     y = 10 - (t-10)^2;
% else
%     y=t;
% end
y = t;
end


function q = psid(t)

% global L1 L2 L3;
% q = 1.32;
q = atan2(yd(t),xd(t));
% q = 1.32;
end

function q = th1d(t)
L0=1.5;L1=0.3;L2=0.3;L3=0.08; % L3 항상 지면에 수직. 
tf=10; w = 10*pi/tf;
% global L1 L2 L3;
% q = -pi/6;
q = atan2(zd(t)-L3-1.5,sqrt(xd(t)^2+yd(t)^2)) - atan2(L2*sin(th2d(t)),L1+L2*cos(th2d(t)));
% q = -1.52;
end

function q = th2d(t)
L0=1.5;L1=0.3;L2=0.3;L3=0.08; % L3 항상 지면에 수직. 
tf=10; w = 10*pi/tf;
% global L1 L2 L3;
% q = pi/3;
q = acos((xd(t)^2 + yd(t)^2 +(zd(t)-L3-1.5)^2-L1^2-L2^2)/(2*L1*L2));
% q = 1.57;
end

function y = th3d(t)
L0=1.5;L1=0.3;L2=0.3;L3=0.08; % L3 항상 지면에 수직. 
tf=10; w = 10*pi/tf;
% global L1 L2 L3;
y = pi/2 - th1d(t) - th2d(t);
% y = 1.52;
end

function y = xd(t)
L0=1.5;L1=0.3;L2=0.3;L3=0.08; % L3 항상 지면에 수직.
scale_factor = 1/80; cycle = 1;
tf=10; w = 2*pi*cycle;
y = scale_factor*(1 + cos(w*s(t)))-4.1750e-04- 1.469294361278199e-06;
% global L1 L2 L3 w tf;
% y = ((10 - (10/tf)*(t))*cos(w*(t)))/100;
% y = ((10 - (10/tf)*s(t))*cos(w*s(t)))/100;
% y = (50*cos(pi/4)+(-2*50*cos(pi/4))*s(t)/tf)/100; % 서빙 to 어피치 
end

function y = yd(t)
L0=1.5;L1=0.3;L2=0.3;L3=0.08; % L3 항상 지면에 수직. 
scale_factor = 1/80; cycle = 1;
tf=10; w = 2*pi*cycle;
y = scale_factor*(-2 + sin(w*s(t))) + 0.4-1.0582e-04+ 0.00000326818465700;
% global L1 L2 L3 w tf;
% y = ((10 - (10/tf)*(t))*sin(w*(t)) + 40)/100;  % (0,40) 에서 sprial sink./*
% y = ((10 - (10/tf)*s(t))*sin(w*s(t)) + 40)/100;  % (0,40) 에서 sprial sink.
% y = (0.7 .* s(t).*(s(t)-10) + 50*sin(pi/4))/100; % 두배가량 내려감
end

function y = zd(t)
L0=1.5;L1=0.3;L2=0.3;L3=0.08; % L3 항상 지면에 수직. 
scale_factor = 1/80; cycle = 1;
tf=10; w = 2*pi*cycle;
y = 1.3+ 0.000013186867988;
end

== matlab function total_senario/Desired Joint Trajectory/MATLAB Function5 ==
  data: u input; qd output

function qd = fcn(u)
t = u(1);
% time = 0:0.01:10

% (1) r_t,theta_t _ // for Tornado
% cycle=5; % 해당 시간동안 몇바퀴 돌지_진동수
% r_t = 0.1 - (0.1/tf)*t; 
% w_t = cycle*2*pi/tf; 
% theta_t = w_t*t;
% 
% % (2) waffle 중심 cartesian coordinate
% x_wa = r_t.*cos(theta_t); % waffle 중심  
% y_wa = r_t.*sin(theta_t) + 0.4;
% z_wa = - 0.2 - (0.3/tf)*t + 0.6; 
% r_wa = sqrt(x_wa.^2+y_wa.^2);

% psii= atan2(y_wa,x_wa);
% th2 = acos((r_wa.^2+z_wa.^2-L1^2-L2^2)./(2*L1*L2)); % r,z 좌표계로 사이드뷰
% th1 = atan2(z_wa-L3,r_wa) - atan2(L2*sin(th2),L1+L2*cos(th2));
% th3 = pi/2-th1-th2;

x = 0;
y = 0.4;

scale_factor = 1/80;
cycle = 1;
time = 1; %% 20
t=t/time;
w = 2*pi*cycle;
theta = w*t;


psii= psid(t);
th2 = th2d(t); % r,z 좌표계로 사이드뷰
th1 = th1d(t);
th3 = th3d(t);


qd = [psii; th1; th2; th3];

end

function y = s(t)
% if (-1<=t && t<3)
%     y = 2/3*t^3 - 8/27*t^4 +1/27*t^5;
% %     y = 3/2*t^3 - 1*t^4 +3/16*t^5; % 5 / 2
% %     y = 6*t^3 -8*t^4 + 3*t^5; % 5차 1초
% %     y = 2/3*t^2-1/9*t^3; % 3초
% %     y = t^2 - 0.25*t^3; % 2초
% %     y = 2*t^2 - t^3; % 1초
% %     y = t^2;
% elseif (3<=t && t<7)
%     y = t;
% elseif (7<=t &&  t<=10.01)
%     y = -37730/27 + 2600/3*t -5740/27*t^2 + 698/27*t^3 -14/9*t^4 + 1/27*t^5;
% %     y = -10240 + 5825*t -1320*t^2 + 149*t^3 -67/8*t^4 + 3/16*t^5; % 5 / 2
% %     y = -225990 + 119800*t -25380*t^2 + 2686*t^3 -142*t^4 + 3*t^5; % 5차1s
% %     y = 490/9 - 20*t + 8/3*t^2 - 1/9*t^3; % 3초
% %     y = 160 - 55*t +6.5 * t^2 - 0.25*t^3; % 2초
% %     y = 810 - 260*t + 28*t^2 - t^3; % 1초
% %     y = 10 - (t-10)^2;
% else
%     y=t;
% end
y = t;
end


function q = psid(t)

% global L1 L2 L3;
% q = 1.32;
q = atan2(yd(t),xd(t));
% q = 1.32;
end

function q = th1d(t)
L0=1.5;L1=0.3;L2=0.3;L3=0.08; % L3 항상 지면에 수직. 
tf=10; w = 10*pi/tf;
% global L1 L2 L3;
% q = -pi/6;
q = atan2(zd(t)-L3-1.5,sqrt(xd(t)^2+yd(t)^2)) - atan2(L2*sin(th2d(t)),L1+L2*cos(th2d(t)));
% q = -1.52;
end

function q = th2d(t)
L0=1.5;L1=0.3;L2=0.3;L3=0.08; % L3 항상 지면에 수직. 
tf=10; w = 10*pi/tf;
% global L1 L2 L3;
% q = pi/3;
q = acos((xd(t)^2 + yd(t)^2 +(zd(t)-L3-1.5)^2-L1^2-L2^2)/(2*L1*L2));
% q = 1.57;
end

function y = th3d(t)
L0=1.5;L1=0.3;L2=0.3;L3=0.08; % L3 항상 지면에 수직. 
tf=10; w = 10*pi/tf;
% global L1 L2 L3;
y = pi/2 - th1d(t) - th2d(t);
% y = 1.52;
end

function y = xd(t)
L0=1.5;L1=0.3;L2=0.3;L3=0.08; % L3 항상 지면에 수직.
scale_factor = 1/80; cycle = 1;
tf=10; w = 2*pi*cycle;
y = scale_factor*0.5*cos(w*s(t))-4.1750e-04 -5.4336e-05- 1.469294361278199e-06;
% global L1 L2 L3 w tf;
% y = ((10 - (10/tf)*(t))*cos(w*(t)))/100;
% y = ((10 - (10/tf)*s(t))*cos(w*s(t)))/100;
% y = (50*cos(pi/4)+(-2*50*cos(pi/4))*s(t)/tf)/100; % 서빙 to 어피치 
end

function y = yd(t)
L0=1.5;L1=0.3;L2=0.3;L3=0.08; % L3 항상 지면에 수직. 
scale_factor = 1/80; cycle = 1;
tf=10; w = 2*pi*cycle;
y = scale_factor*(-1 + 0.5*sin(w*s(t))) + 0.4-1.0582e-04 + 3.6226e-05+ 0.00000326818465700;
% global L1 L2 L3 w tf;
% y = ((10 - (10/tf)*(t))*sin(w*(t)) + 40)/100;  % (0,40) 에서 sprial sink./*
% y = ((10 - (10/tf)*s(t))*sin(w*s(t)) + 40)/100;  % (0,40) 에서 sprial sink.
% y = (0.7 .* s(t).*(s(t)-10) + 50*sin(pi/4))/100; % 두배가량 내려감
end

function y = zd(t)
L0=1.5;L1=0.3;L2=0.3;L3=0.08; % L3 항상 지면에 수직. 
scale_factor = 1/80; cycle = 1;
tf=10; w = 2*pi*cycle;
y = 1.3+ 0.000013186867988;
end

== matlab function total_senario/Desired Joint Trajectory/MATLAB Function6 ==
  data: u input; qd output

function qd = fcn(u)
t = u(1);
% time = 0:0.01:10

% (1) r_t,theta_t _ // for Tornado
% cycle=5; % 해당 시간동안 몇바퀴 돌지_진동수
% r_t = 0.1 - (0.1/tf)*t; 
% w_t = cycle*2*pi/tf; 
% theta_t = w_t*t;
% 
% % (2) waffle 중심 cartesian coordinate
% x_wa = r_t.*cos(theta_t); % waffle 중심  
% y_wa = r_t.*sin(theta_t) + 0.4;
% z_wa = - 0.2 - (0.3/tf)*t + 0.6; 
% r_wa = sqrt(x_wa.^2+y_wa.^2);

% psii= atan2(y_wa,x_wa);
% th2 = acos((r_wa.^2+z_wa.^2-L1^2-L2^2)./(2*L1*L2)); % r,z 좌표계로 사이드뷰
% th1 = atan2(z_wa-L3,r_wa) - atan2(L2*sin(th2),L1+L2*cos(th2));
% th3 = pi/2-th1-th2;

x = 0;
y = 0.4;

scale_factor = 1/80;
cycle = 1;
time = 1; %% 20
t=t/time;
w = 2*pi*cycle;
theta = w*t;


psii= psid(t);
th2 = th2d(t); % r,z 좌표계로 사이드뷰
th1 = th1d(t);
th3 = th3d(t);


qd = [psii; th1; th2; th3];

end

function y = s(t)
% if (-1<=t && t<3)
%     y = 2/3*t^3 - 8/27*t^4 +1/27*t^5;
% %     y = 3/2*t^3 - 1*t^4 +3/16*t^5; % 5 / 2
% %     y = 6*t^3 -8*t^4 + 3*t^5; % 5차 1초
% %     y = 2/3*t^2-1/9*t^3; % 3초
% %     y = t^2 - 0.25*t^3; % 2초
% %     y = 2*t^2 - t^3; % 1초
% %     y = t^2;
% elseif (3<=t && t<7)
%     y = t;
% elseif (7<=t &&  t<=10.01)
%     y = -37730/27 + 2600/3*t -5740/27*t^2 + 698/27*t^3 -14/9*t^4 + 1/27*t^5;
% %     y = -10240 + 5825*t -1320*t^2 + 149*t^3 -67/8*t^4 + 3/16*t^5; % 5 / 2
% %     y = -225990 + 119800*t -25380*t^2 + 2686*t^3 -142*t^4 + 3*t^5; % 5차1s
% %     y = 490/9 - 20*t + 8/3*t^2 - 1/9*t^3; % 3초
% %     y = 160 - 55*t +6.5 * t^2 - 0.25*t^3; % 2초
% %     y = 810 - 260*t + 28*t^2 - t^3; % 1초
% %     y = 10 - (t-10)^2;
% else
%     y=t;
% end
y = t;
end


function q = psid(t)

% global L1 L2 L3;
% q = 1.32;
q = atan2(yd(t),xd(t));
% q = 1.32;
end

function q = th1d(t)
L0=1.5;L1=0.3;L2=0.3;L3=0.08; % L3 항상 지면에 수직. 
tf=10; w = 10*pi/tf;
% global L1 L2 L3;
% q = -pi/6;
q = atan2(zd(t)-L3-1.5,sqrt(xd(t)^2+yd(t)^2)) - atan2(L2*sin(th2d(t)),L1+L2*cos(th2d(t)));
% q = -1.52;
end

function q = th2d(t)
L0=1.5;L1=0.3;L2=0.3;L3=0.08; % L3 항상 지면에 수직. 
tf=10; w = 10*pi/tf;
% global L1 L2 L3;
% q = pi/3;
q = acos((xd(t)^2 + yd(t)^2 +(zd(t)-L3-1.5)^2-L1^2-L2^2)/(2*L1*L2));
% q = 1.57;
end

function y = th3d(t)
L0=1.5;L1=0.3;L2=0.3;L3=0.08; % L3 항상 지면에 수직. 
tf=10; w = 10*pi/tf;
% global L1 L2 L3;
y = pi/2 - th1d(t) - th2d(t);
% y = 1.52;
end

function y = xd(t)
L0=1.5;L1=0.3;L2=0.3;L3=0.08; % L3 항상 지면에 수직.
scale_factor = 1/80; cycle = 1;
tf=10; w = 2*pi*cycle;
y = scale_factor*(3 + cos(w*s(t)))-4.1750e-04 -4.3728e-05- 1.469294361278199e-06;
% global L1 L2 L3 w tf;
% y = ((10 - (10/tf)*(t))*cos(w*(t)))/100;
% y = ((10 - (10/tf)*s(t))*cos(w*s(t)))/100;
% y = (50*cos(pi/4)+(-2*50*cos(pi/4))*s(t)/tf)/100; % 서빙 to 어피치 
end

function y = yd(t)
L0=1.5;L1=0.3;L2=0.3;L3=0.08; % L3 항상 지면에 수직. 
scale_factor = 1/80; cycle = 1;
tf=10; w = 2*pi*cycle;
y = scale_factor*(1 + sin(w*s(t))) + 0.4-1.0582e-04 + 3.9610e-05+ 0.00000326818465700; 
% global L1 L2 L3 w tf;
% y = ((10 - (10/tf)*(t))*sin(w*(t)) + 40)/100;  % (0,40) 에서 sprial sink./*
% y = ((10 - (10/tf)*s(t))*sin(w*s(t)) + 40)/100;  % (0,40) 에서 sprial sink.
% y = (0.7 .* s(t).*(s(t)-10) + 50*sin(pi/4))/100; % 두배가량 내려감
end

function y = zd(t)
L0=1.5;L1=0.3;L2=0.3;L3=0.08; % L3 항상 지면에 수직. 
scale_factor = 1/80; cycle = 1;
tf=10; w = 2*pi*cycle;
y = 1.3+ 0.000013186867988;
end

== matlab function total_senario/Desired Joint Trajectory/MATLAB Function7 ==
  data: u input; qd output

function qd = fcn(u)
t = u(1);
% time = 0:0.01:10

% (1) r_t,theta_t _ // for Tornado
% cycle=5; % 해당 시간동안 몇바퀴 돌지_진동수
% r_t = 0.1 - (0.1/tf)*t; 
% w_t = cycle*2*pi/tf; 
% theta_t = w_t*t;
% 
% % (2) waffle 중심 cartesian coordinate
% x_wa = r_t.*cos(theta_t); % waffle 중심  
% y_wa = r_t.*sin(theta_t) + 0.4;
% z_wa = - 0.2 - (0.3/tf)*t + 0.6; 
% r_wa = sqrt(x_wa.^2+y_wa.^2);

% psii= atan2(y_wa,x_wa);
% th2 = acos((r_wa.^2+z_wa.^2-L1^2-L2^2)./(2*L1*L2)); % r,z 좌표계로 사이드뷰
% th1 = atan2(z_wa-L3,r_wa) - atan2(L2*sin(th2),L1+L2*cos(th2));
% th3 = pi/2-th1-th2;

x = 0;
y = 0.4;

scale_factor = 1/80;
cycle = 1;
time = 1; %% 20
t=t/time;
w = 2*pi*cycle;
theta = w*t;


psii= psid(t);
th2 = th2d(t); % r,z 좌표계로 사이드뷰
th1 = th1d(t);
th3 = th3d(t);


qd = [psii; th1; th2; th3];

end

function y = s(t)
% if (-1<=t && t<3)
%     y = 2/3*t^3 - 8/27*t^4 +1/27*t^5;
% %     y = 3/2*t^3 - 1*t^4 +3/16*t^5; % 5 / 2
% %     y = 6*t^3 -8*t^4 + 3*t^5; % 5차 1초
% %     y = 2/3*t^2-1/9*t^3; % 3초
% %     y = t^2 - 0.25*t^3; % 2초
% %     y = 2*t^2 - t^3; % 1초
% %     y = t^2;
% elseif (3<=t && t<7)
%     y = t;
% elseif (7<=t &&  t<=10.01)
%     y = -37730/27 + 2600/3*t -5740/27*t^2 + 698/27*t^3 -14/9*t^4 + 1/27*t^5;
% %     y = -10240 + 5825*t -1320*t^2 + 149*t^3 -67/8*t^4 + 3/16*t^5; % 5 / 2
% %     y = -225990 + 119800*t -25380*t^2 + 2686*t^3 -142*t^4 + 3*t^5; % 5차1s
% %     y = 490/9 - 20*t + 8/3*t^2 - 1/9*t^3; % 3초
% %     y = 160 - 55*t +6.5 * t^2 - 0.25*t^3; % 2초
% %     y = 810 - 260*t + 28*t^2 - t^3; % 1초
% %     y = 10 - (t-10)^2;
% else
%     y=t;
% end
y = t;
end


function q = psid(t)

% global L1 L2 L3;
% q = 1.32;
q = atan2(yd(t),xd(t));
% q = 1.32;
end

function q = th1d(t)
L0=1.5;L1=0.3;L2=0.3;L3=0.08; % L3 항상 지면에 수직. 
tf=10; w = 10*pi/tf;
% global L1 L2 L3;
% q = -pi/6;
q = atan2(zd(t)-L3-1.5,sqrt(xd(t)^2+yd(t)^2)) - atan2(L2*sin(th2d(t)),L1+L2*cos(th2d(t)));
% q = -1.52;
end

function q = th2d(t)
L0=1.5;L1=0.3;L2=0.3;L3=0.08; % L3 항상 지면에 수직. 
tf=10; w = 10*pi/tf;
% global L1 L2 L3;
% q = pi/3;
q = acos((xd(t)^2 + yd(t)^2 +(zd(t)-L3-1.5)^2-L1^2-L2^2)/(2*L1*L2));
% q = 1.57;
end

function y = th3d(t)
L0=1.5;L1=0.3;L2=0.3;L3=0.08; % L3 항상 지면에 수직. 
tf=10; w = 10*pi/tf;
% global L1 L2 L3;
y = pi/2 - th1d(t) - th2d(t);
% y = 1.52;
end

function y = xd(t)
L0=1.5;L1=0.3;L2=0.3;L3=0.08; % L3 항상 지면에 수직.
scale_factor = 1/80; cycle = 1;
tf=10; w = 2*pi*cycle;
y = scale_factor*(-3 + cos(w*s(t)))-4.1750e-04 + 4.3728e-05 -8.7456e-05- 1.469294361278199e-06;
% global L1 L2 L3 w tf;
% y = ((10 - (10/tf)*(t))*cos(w*(t)))/100;
% y = ((10 - (10/tf)*s(t))*cos(w*s(t)))/100;
% y = (50*cos(pi/4)+(-2*50*cos(pi/4))*s(t)/tf)/100; % 서빙 to 어피치 
end

function y = yd(t)
L0=1.5;L1=0.3;L2=0.3;L3=0.08; % L3 항상 지면에 수직. 
scale_factor = 1/80; cycle = 1;
tf=10; w = 2*pi*cycle;
y = scale_factor*(1 + sin(w*s(t))) + 0.4-1.0582e-04+3.9610e-05+ 0.00000326818465700;
% global L1 L2 L3 w tf;
% y = ((10 - (10/tf)*(t))*sin(w*(t)) + 40)/100;  % (0,40) 에서 sprial sink./*
% y = ((10 - (10/tf)*s(t))*sin(w*s(t)) + 40)/100;  % (0,40) 에서 sprial sink.
% y = (0.7 .* s(t).*(s(t)-10) + 50*sin(pi/4))/100; % 두배가량 내려감
end

function y = zd(t)
L0=1.5;L1=0.3;L2=0.3;L3=0.08; % L3 항상 지면에 수직. 
scale_factor = 1/80; cycle = 1;
tf=10; w = 2*pi*cycle;
y = 1.3+ 0.000013186867988;
end

== matlab function total_senario/Desired Joint Trajectory/MATLAB Function8 ==
  data: u input; qd output

function qd = fcn(u)
t = u(1);


psii= psid(t);
th2 = th2d(t); % r,z 좌표계로 사이드뷰
th1 = th1d(t);
th3 = th3d(t);

qd = [psii; th1; th2; th3];
end


function q = psid(t)

if -1<=t && t<0.9759
    q = 11781/5000 - t^2/10;
elseif 0.9759<=t && t<4.0241
    q = 17250406981767201526670181/7036874417766400000000000 - (1757953092946309*t)/9007199254740992;
elseif 4.0241<=t && t<=6
    q = (t - 1132695502984799/281474976710656)^2/10 - (1757953092946309*t)/9007199254740992 + 17250406981767201526670181/7036874417766400000000000;
else
    q = 0;
end

end

function q = th1d(t)
if -1<=t && t<0.5713
    q = - t^2/10 - 7249/10000;
elseif 0.5713<=t && t<4.4287
    q = - (4116434174604709*t)/36028797018963968 - 38971058255599631882930373/56294995342131200000000000;
elseif 4.4287<=t && t<=6
    q = (t - 4986305537332329/1125899906842624)^2/10 - (4116434174604709*t)/36028797018963968 - 38971058255599631882930373/56294995342131200000000000;
else
    q = 0;
end



end

function q = th2d(t)
if -1<=t && t<0.1104
    q = t^2/10 + 2831/2500;
elseif 0.1104<=t && t<4.8895
    q = (6366432548439009*t)/288230376151711744 + 127359579511278740948711439/112589990684262400000000000;
elseif 4.8895<=t && t<=6
    q = (6366432548439009*t)/288230376151711744 - (t - 13500/2761)^2/10 + 127359579511278740948711439/112589990684262400000000000;
else
    q = 0;
end
end

function y = th3d(t)
y = pi/2 - th1d(t) - th2d(t);
end

== matlab function total_senario/Desired Joint Trajectory/MATLAB Function9 ==
  data: u input; qd output

function qd = fcn(u)
t = u(1);
% time = 0:0.01:10

% (1) r_t,theta_t _ // for Tornado
% cycle=5; % 해당 시간동안 몇바퀴 돌지_진동수
% r_t = 0.1 - (0.1/tf)*t; 
% w_t = cycle*2*pi/tf; 
% theta_t = w_t*t;
% 
% % (2) waffle 중심 cartesian coordinate
% x_wa = r_t.*cos(theta_t); % waffle 중심  
% y_wa = r_t.*sin(theta_t) + 0.4;
% z_wa = - 0.2 - (0.3/tf)*t + 0.6; 
% r_wa = sqrt(x_wa.^2+y_wa.^2);

% psii= atan2(y_wa,x_wa);
% th2 = acos((r_wa.^2+z_wa.^2-L1^2-L2^2)./(2*L1*L2)); % r,z 좌표계로 사이드뷰
% th1 = atan2(z_wa-L3,r_wa) - atan2(L2*sin(th2),L1+L2*cos(th2));
% th3 = pi/2-th1-th2;

x = 0;
y = 0.4;

scale_factor = 1/80;
cycle = 1;
time = 1; %% 20
t=t/time;
w = 2*pi*cycle;
theta = w*t;


psii= psid(t);
th2 = th2d(t); % r,z 좌표계로 사이드뷰
th1 = th1d(t);
th3 = th3d(t);


qd = [psii; th1; th2; th3];

end

function y = s(t)
% if (-1<=t && t<3)
%     y = 2/3*t^3 - 8/27*t^4 +1/27*t^5;
% %     y = 3/2*t^3 - 1*t^4 +3/16*t^5; % 5 / 2
% %     y = 6*t^3 -8*t^4 + 3*t^5; % 5차 1초
% %     y = 2/3*t^2-1/9*t^3; % 3초
% %     y = t^2 - 0.25*t^3; % 2초
% %     y = 2*t^2 - t^3; % 1초
% %     y = t^2;
% elseif (3<=t && t<7)
%     y = t;
% elseif (7<=t &&  t<=10.01)
%     y = -37730/27 + 2600/3*t -5740/27*t^2 + 698/27*t^3 -14/9*t^4 + 1/27*t^5;
% %     y = -10240 + 5825*t -1320*t^2 + 149*t^3 -67/8*t^4 + 3/16*t^5; % 5 / 2
% %     y = -225990 + 119800*t -25380*t^2 + 2686*t^3 -142*t^4 + 3*t^5; % 5차1s
% %     y = 490/9 - 20*t + 8/3*t^2 - 1/9*t^3; % 3초
% %     y = 160 - 55*t +6.5 * t^2 - 0.25*t^3; % 2초
% %     y = 810 - 260*t + 28*t^2 - t^3; % 1초
% %     y = 10 - (t-10)^2;
% else
%     y=t;
% end
y = t;
end


function q = psid(t)

% global L1 L2 L3;
% q = 1.32;
q = atan2(yd(t),xd(t));
% q = 1.32;
end

function q = th1d(t)
L0=1.5;L1=0.3;L2=0.3;L3=0.08; % L3 항상 지면에 수직. 
tf=10; w = 10*pi/tf;
% global L1 L2 L3;
% q = -pi/6;
q = atan2(zd(t)-L3-1.5,sqrt(xd(t)^2+yd(t)^2)) - atan2(L2*sin(th2d(t)),L1+L2*cos(th2d(t)));
% q = -1.52;
end

function q = th2d(t)
L0=1.5;L1=0.3;L2=0.3;L3=0.08; % L3 항상 지면에 수직. 
tf=10; w = 10*pi/tf;
% global L1 L2 L3;
% q = pi/3;
q = acos((xd(t)^2 + yd(t)^2 +(zd(t)-L3-1.5)^2-L1^2-L2^2)/(2*L1*L2));
% q = 1.57;
end

function y = th3d(t)
L0=1.5;L1=0.3;L2=0.3;L3=0.08; % L3 항상 지면에 수직. 
tf=10; w = 10*pi/tf;
% global L1 L2 L3;
y = pi/2 - th1d(t) - th2d(t);
% y = 1.52;
end

function y = xd(t)
L0=1.5;L1=0.3;L2=0.3;L3=0.08; % L3 항상 지면에 수직.
scale_factor = 1/80; cycle = 1;
tf=10; w = 2*pi*cycle;
y = -0.0125+0.013975*cos(0.5*w*t+2.67794+pi)- 1.469294361278199e-06-4.616395336579059e-04;
% global L1 L2 L3 w tf;
% y = ((10 - (10/tf)*(t))*cos(w*(t)))/100;
% y = ((10 - (10/tf)*s(t))*cos(w*s(t)))/100;
% y = (50*cos(pi/4)+(-2*50*cos(pi/4))*s(t)/tf)/100; % 서빙 to 어피치 
end

function y = yd(t)
L0=1.5;L1=0.3;L2=0.3;L3=0.08; % L3 항상 지면에 수직. 
scale_factor = 1/80; cycle = 1;
tf=10; w = 2*pi*cycle;
y =  0.40625 + 0.013975*sin(0.5*w*t+2.67794+pi)+ 0.00000326818465700-6.608305247779445e-05;
% global L1 L2 L3 w tf;
% y = ((10 - (10/tf)*(t))*sin(w*(t)) + 40)/100;  % (0,40) 에서 sprial sink./*
% y = ((10 - (10/tf)*s(t))*sin(w*s(t)) + 40)/100;  % (0,40) 에서 sprial sink.
% y = (0.7 .* s(t).*(s(t)-10) + 50*sin(pi/4))/100; % 두배가량 내려감
end

function y = zd(t)
L0=1.5;L1=0.3;L2=0.3;L3=0.08; % L3 항상 지면에 수직. 
scale_factor = 1/80; cycle = 1;
tf=10; w = 2*pi*cycle;
y = 1.3+ 0.000013186867988;
end

== matlab function total_senario/Desired Joint Trajectory/MATLAB Function10 ==
  data: t input; qd output; a input; b input; c input
function qd = fcn(t, a, b, c)
% qd = zeros(4, 1);
qd = 0;
check = 0;
d =4;

if (t < 1)
    check = a
    
elseif ( (t < 2))
    check = b
    
elseif ((t < 3))
    check = c
else
    check = d
end
qd = check;
end

== matlab function total_senario/Desired Joint Trajectory/MATLAB Function11 ==
  data: u input; qd output

function qd = fcn(u)
t = u(1);
% time = 0:0.01:10

% (1) r_t,theta_t _ // for Tornado
% cycle=5; % 해당 시간동안 몇바퀴 돌지_진동수
% r_t = 0.1 - (0.1/tf)*t; 
% w_t = cycle*2*pi/tf; 
% theta_t = w_t*t;
% 
% % (2) waffle 중심 cartesian coordinate
% x_wa = r_t.*cos(theta_t); % waffle 중심  
% y_wa = r_t.*sin(theta_t) + 0.4;
% z_wa = - 0.2 - (0.3/tf)*t + 0.6; 
% r_wa = sqrt(x_wa.^2+y_wa.^2);

% psii= atan2(y_wa,x_wa);
% th2 = acos((r_wa.^2+z_wa.^2-L1^2-L2^2)./(2*L1*L2)); % r,z 좌표계로 사이드뷰
% th1 = atan2(z_wa-L3,r_wa) - atan2(L2*sin(th2),L1+L2*cos(th2));
% th3 = pi/2-th1-th2;

x = 0;
y = 0.4;

scale_factor = 1/80;
cycle = 1;
time = 1; %% 20
t=t/time;
w = 2*pi*cycle;
theta = w*t;


psii= psid(t);
th2 = th2d(t); % r,z 좌표계로 사이드뷰
th1 = th1d(t);
th3 = th3d(t);


qd = [psii; th1; th2; th3];

end

function y = s(t)
% if (-1<=t && t<3)
%     y = 2/3*t^3 - 8/27*t^4 +1/27*t^5;
% %     y = 3/2*t^3 - 1*t^4 +3/16*t^5; % 5 / 2
% %     y = 6*t^3 -8*t^4 + 3*t^5; % 5차 1초
% %     y = 2/3*t^2-1/9*t^3; % 3초
% %     y = t^2 - 0.25*t^3; % 2초
% %     y = 2*t^2 - t^3; % 1초
% %     y = t^2;
% elseif (3<=t && t<7)
%     y = t;
% elseif (7<=t &&  t<=10.01)
%     y = -37730/27 + 2600/3*t -5740/27*t^2 + 698/27*t^3 -14/9*t^4 + 1/27*t^5;
% %     y = -10240 + 5825*t -1320*t^2 + 149*t^3 -67/8*t^4 + 3/16*t^5; % 5 / 2
% %     y = -225990 + 119800*t -25380*t^2 + 2686*t^3 -142*t^4 + 3*t^5; % 5차1s
% %     y = 490/9 - 20*t + 8/3*t^2 - 1/9*t^3; % 3초
% %     y = 160 - 55*t +6.5 * t^2 - 0.25*t^3; % 2초
% %     y = 810 - 260*t + 28*t^2 - t^3; % 1초
% %     y = 10 - (t-10)^2;
% else
%     y=t;
% end
y = t;
end


function q = psid(t)

% global L1 L2 L3;
% q = 1.32;
q = atan2(yd(t),xd(t));
% q = 1.32;
end

function q = th1d(t)
L0=1.5;L1=0.3;L2=0.3;L3=0.08; % L3 항상 지면에 수직. 
tf=10; w = 10*pi/tf;
% global L1 L2 L3;
% q = -pi/6;
q = atan2(zd(t)-L3-1.5,sqrt(xd(t)^2+yd(t)^2)) - atan2(L2*sin(th2d(t)),L1+L2*cos(th2d(t)));
% q = -1.52;
end

function q = th2d(t)
L0=1.5;L1=0.3;L2=0.3;L3=0.08; % L3 항상 지면에 수직. 
tf=10; w = 10*pi/tf;
% global L1 L2 L3;
% q = pi/3;
q = acos((xd(t)^2 + yd(t)^2 +(zd(t)-L3-1.5)^2-L1^2-L2^2)/(2*L1*L2));
% q = 1.57;
end

function y = th3d(t)
L0=1.5;L1=0.3;L2=0.3;L3=0.08; % L3 항상 지면에 수직. 
tf=10; w = 10*pi/tf;
% global L1 L2 L3;
y = pi/2 - th1d(t) - th2d(t);
% y = 1.52;
end

function y = xd(t)
L0=1.5;L1=0.3;L2=0.3;L3=0.08; % L3 항상 지면에 수직.
scale_factor = 1/80; cycle = 1;
tf=10; w = 2*pi*cycle;
y = 0.09375+0.038*cos(0.5*w*t+pi-1.4)- 1.469294361278199e-06 -0.00020875;
% global L1 L2 L3 w tf;
% y = ((10 - (10/tf)*(t))*cos(w*(t)))/100;
% y = ((10 - (10/tf)*s(t))*cos(w*s(t)))/100;
% y = (50*cos(pi/4)+(-2*50*cos(pi/4))*s(t)/tf)/100; % 서빙 to 어피치 
end

function y = yd(t)
L0=1.5;L1=0.3;L2=0.3;L3=0.08; % L3 항상 지면에 수직. 
scale_factor = 1/80; cycle = 1;
tf=10; w = 2*pi*cycle;
y = 0.4375+0.038*sin(0.5*w*t+pi-1.4)+ 0.00000326818465700-0.00005291;
% global L1 L2 L3 w tf;
% y = ((10 - (10/tf)*(t))*sin(w*(t)) + 40)/100;  % (0,40) 에서 sprial sink./*
% y = ((10 - (10/tf)*s(t))*sin(w*s(t)) + 40)/100;  % (0,40) 에서 sprial sink.
% y = (0.7 .* s(t).*(s(t)-10) + 50*sin(pi/4))/100; % 두배가량 내려감
end

function y = zd(t)
L0=1.5;L1=0.3;L2=0.3;L3=0.08; % L3 항상 지면에 수직. 
scale_factor = 1/80; cycle = 1;
tf=10; w = 2*pi*cycle;
y = 1.3+ 0.000013186867988;
end

== matlab function total_senario/Desired Joint Trajectory/MATLAB Function12 ==
  data: u input; y output
function y = fcn(u)
t = u(1);
if t<9
    y = 9;
elseif (t<10)
    y = t;
else
    y=10;
end
 
    
end
